simulink model "Kalman_Fliter"  (R2022b)
settings: Solver=VariableStepAuto  StartTime=0.0  StopTime=30  RelTol=1e-3
libraries: dspmathops x1
settings Model: Creator=zhouwenjie  LastModifiedBy=zhouwenjie

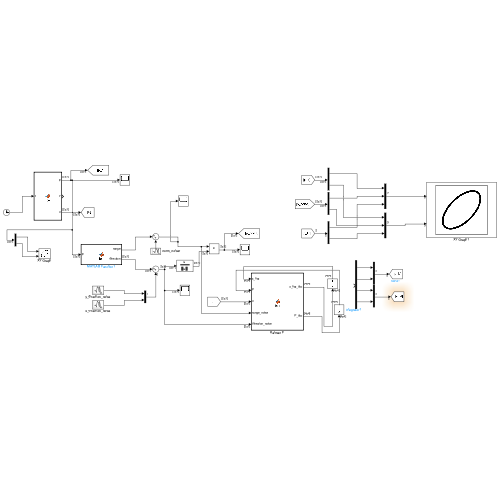
[thumbnail: Simulink's stored preview of the top-level diagram]
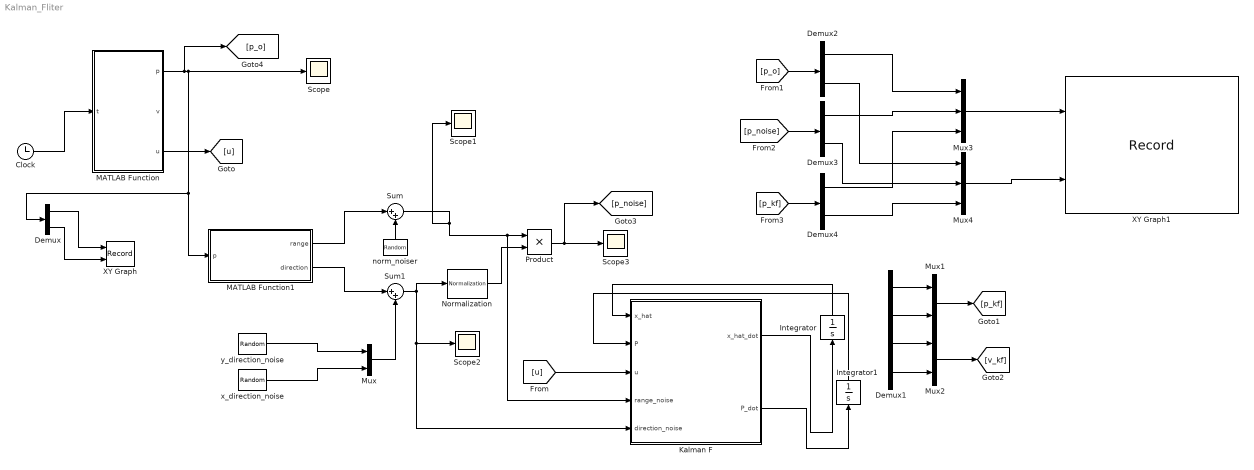
== system Kalman_Fliter ==
  Clock : Clock
  Demux{,2..4} (4 alike) : Demux  Outputs=2
  Demux1 : Demux
  Integrator : Integrator
  Integrator1 : Integrator
  Kalman F : MATLAB Function  TreatAsAtomicUnit=on
  MATLAB Function : MATLAB Function  TreatAsAtomicUnit=on
  MATLAB Function1 : MATLAB Function  TreatAsAtomicUnit=on
  Mux : Mux  Inputs=2
  Mux1 : Mux  Inputs=2
  Mux2 : Mux  Inputs=2
  Mux3 : Mux  Inputs=3
  Mux4 : Mux  Inputs=3
  Normalization : dspmathops/Normalization  NormType=2-norm  Bias=1e-10  NormOver=Each column  Dimension=1  roundingMode=Floor  overflowMode=off  accumDataTypeStr=Inherit: Same as product output  accumLastDataTypeStr=Inherit: Same as product output  outputDataTypeStr=Inherit: Same as product output  outputMin=[]  outputMax=[]  outputLastDataTypeStr=Inherit: Same as product output
  Product : Product
  Scope{,1..3} (4 alike) : Scope
  Sum : Sum  Inputs=|++
  Sum1 : Sum  Inputs=|++
  XY Graph : Record  FileSettingsInternal="{\"entries\":[{\"content\":{\"excelSettings\":{\"content\":{},\"type\":\"Streamout.ExcelSettings\"}},\"type\":\"Streamout.FileSettingStorage\",\"uuid\":\"d119d5ed-e209-42ba-8edb-009befcb7634\"}],\"packageUris\":[\"http://schema.mathworks.com/mf0/streamout_blocks/R2020a\"],\"version\":\"1.0\"}"  Layout=[1 1]  SignalsInternal="{\"entries\":[{\"content\":{\"signals\":[{\"content\":{\"blockPath\":[\"Kalman_Fliter/XY Graph\"],\"channel\":[],\"dimensions\":[1,1],\"domain\":\"Kalman_Fliter/XY Graph\",\"lineColor\":\"#a2142f\",\"plots\":[1],\"port\":1,\"sid\":[\"\"],\"signalID\":563,\"signalName\":\"Demux:1\"},\"type\":\"RecordBlkView.Signal\",\"uuid\":\"1961980f-dccb-4910-a77f-37722e977325\"},{\"content\":{\"blockPath\":[\"Kalman_Fliter/XY Graph\"],\"channel\":[],\"dimensions\":[1,1],\"domain\":\"Kalman_Fliter/XY Graph\",\"lineColor\":\"#139fff\",\"plots\":[1],\"port\":2,\"sid\":[\"\"],\"signalID\":567,\"signalName\":\"Demux:2\"},\"type\":\"RecordBlkView.Signal\",\"uuid\":\"f8809605-92a7-48fe-8c9b-7ed229beba8b\"}]},\"type\":\"RecordBlkView.InputSignals\",\"uuid\":\"e8c07406-b687-4a26-805d-c1320ae853b1\"}],\"packageUris\":[\"http://schema.mathworks.com/mf0/streamout_blocks/R2020a\"],\"version\":\"1.0\"}"  VisualizationBindings="{\"xyplotplugin\":{\"info\":[{\"series\":[{\"bindingParametersList\":[{\"parameter\":\"X-Axis\",\"signalID\":563,\"signalName\":\"Demux:1\"},{\"parameter\":\"Y-Axis\",\"signalID\":567,\"signalName\":\"Demux:2\"}],\"seriesID\":503},{\"bindingParametersList\":[{\"parameter\":\"Y-Axis\",\"signalID\":567,\"signalName\":\"Demux:2\"},{\"parameter\":\"X-Axis\",\"signalID\":563,\"signalName\":\"Demux:1\"}],\"seriesID\":363}],\"subplotID\":1}]}}"  CompatibilityTag=XY
  XY Graph1 : Record  FileSettingsInternal="{\"entries\":[{\"content\":{\"excelSettings\":{\"content\":{},\"type\":\"Streamout.ExcelSettings\"}},\"type\":\"Streamout.FileSettingStorage\",\"uuid\":\"eefeb38a-37b1-42c2-865b-dc8e865e0e60\"}],\"packageUris\":[\"http://schema.mathworks.com/mf0/streamout_blocks/R2020a\"],\"version\":\"1.0\"}"  Layout=[1 1]  SignalsInternal="{\"entries\":[{\"content\":{\"signals\":[{\"content\":{\"blockPath\":[\"Kalman_Fliter/XY Graph1\"],\"channel\":[],\"dimensions\":[3],\"domain\":\"Kalman_Fliter/XY Graph1\",\"hasChildren\":true,\"lineColor\":\"#64d413\",\"plots\":[],\"port\":1,\"sid\":[\"\"],\"signalID\":571,\"signalName\":\"Mux3\"},\"type\":\"RecordBlkView.Signal\",\"uuid\":\"0d81fedb-c315-4810-a6c0-24634af0a88d\"},{\"content\":{\"blockPath\":[\"Kalman_Fliter/XY Graph1\"],\"channel\":[1],\"dimensions\":[3],\"domain\":\"Kalman_Fliter/XY Graph1\",\"lineColor\":\"#d95319\",\"parentID\":571,\"plots\":[],\"port\":1,\"sid\":[\"\"],\"signalID\":572,\"signalName\":\"Mux3\"},\"type\":\"RecordBlkView.Signal\",\"uuid\":\"11839326-3698-4c45-9993-6f57091d2d65\"},{\"content\":{\"blockPath\":[\"Kalman_Fliter/XY Graph1\"],\"channel\":[],\"dimensions\":[3],\"domain\":\"Kalman_Fliter/XY Graph1\",\"hasChildren\":true,\"lineColor\":\"#fe330a\",\"plots\":[],\"port\":2,\"sid\":[\"\"],\"signalID\":576,\"signalName\":\"Mux4\"},\"type\":\"RecordBlkView.Signal\",\"uuid\":\"38af830b-27b1-40c6-b5d0-badb30e50f9a\"},{\"content\":{\"blockPath\":[\"Kalman_Fliter/XY Graph1\"],\"channel\":[1],\"dimensions\":[3],\"domain\":\"Kalman_Fliter/XY Graph1\",\"lineColor\":\"#7e2f8e\",\"parentID\":576,\"plots\":[],\"port\":2,\"sid\":[\"\"],\"signalID\":577,\"signalName\":\"Mux4\"},\"type\":\"RecordBlkView.Signal\",\"uuid\":\"8c4516df-ef14-4136-9417-f3e6a420cddc\"},{\"content\":{\"blockPath\":[\"Kalman_Fliter/XY Graph1\"],\"channel\":[2],\"dimensions\":[3],\"domain\":\"Kalman_Fliter/XY Graph1\",\"lineColor\":\"#77ac30\",\"parentID\":571,\"plots\":[],\"port\":1,\"sid\":[\"\"],\"signalID\":581,\"signalName\":\"Mux3\"},\"type\":\"RecordBlkView.Signal\",\"uuid\":\"d887d16f-7e2d-4d86-99dc-17678c9a946d\"},{\"content\":{\"blockPath\":[\"Kalman_Fliter/XY Graph1\"],\"channel\":[3],\"dimensions\":[3],\"domain\":\"Kalman_Fliter/XY Graph1\",\"lineColor\":\"#4dbeee\",\"parentID\":571,\"plots\":[],\"port\":1,\"sid\":[\"\"],\"signalID\":582,\"signalName\":\"Mux3\"},\"type\":\"RecordBlkView.Signal\",\"uuid\":\"1185f293-7a12-4181-bfa4-f7e996d1777d\"},{\"content\":{\"blockPath\":[\"Kalman_Fliter/XY Graph1\"],\"channel\":[2],\"dimensions\":[3],\"domain\":\"Kalman_Fliter/XY Graph1\",\"lineColor\":\"#a2142f\",\"parentID\":576,\"plots\":[],\"port\":2,\"sid\":[\"\"],\"signalID\":583,\"signalName\":\"Mux4\"},\"type\":\"RecordBlkView.Signal\",\"uuid\":\"4d6cb4ea-8538-4e3f-b0d2-57ebaadc180e\"},{\"content\":{\"blockPath\":[\"Kalman_Fliter/XY Graph1\"],\"channel\":[3],\"dimensions\":[3],\"domain\":\"Kalman_Fliter/XY Graph1\",\"lineColor\":\"#139fff\",\"parentID\":576,\"plots\":[],\"port\":2,\"sid\":[\"\"],\"signalID\":584,\"signalName\":\"Mux4\"},\"type\":\"RecordBlkView.Signal\",\"uuid\":\"043a01ad-2742-4b7c-882e-cd2255d83c8f\"}]},\"type\":\"RecordBlkView.InputSignals\",\"uuid\":\"c6b6343b-feff-4232-9459-ff0579f05e53\"}],\"packageUris\":[\"http://schema.mathworks.com/mf0/streamout_blocks/R2020a\"],\"version\":\"1.0\"}"  VisualizationBindings="{\"xyplotplugin\":{\"info\":[{\"series\":[],\"subplotID\":1}]}}"  CompatibilityTag=XY
  norm_noiser : RandomNumber  Variance=0.001  SampleTime=0.005
  x_direction_noise : RandomNumber  Variance=0.001  SampleTime=0.005
  y_direction_noise : RandomNumber  Variance=0.001  SampleTime=0.005
  wires:
  Clock/1 -> MATLAB Function/1(t)
  MATLAB Function/1(p) -> [p_o], Demux/1, MATLAB Function1/1(p), Scope/1
  norm_noiser/1 -> Sum/2
  MATLAB Function1/1(range) -> Sum/1
  Sum/1 -> Scope1/1, Kalman F/4(range_noise), Product/1
  MATLAB Function1/2(direction) -> Sum1/1
  y_direction_noise/1 -> Mux/1
  x_direction_noise/1 -> Mux/2
  Mux/1 -> Sum1/2
  Sum1/1 -> Normalization/1, Kalman F/5(direction_noise), Scope2/1
  Demux/1 -> XY Graph/1
  Demux/2 -> XY Graph/2
  Product/1 -> [p_noise], Scope3/1
  Normalization/1 -> Product/2
  [u] -> Kalman F/3(u)
  MATLAB Function/3(u) -> [u]
  Kalman F/2(P_dot) -> Integrator1/1
  Kalman F/1(x_hat_dot) -> Integrator/1
  Integrator1/1 -> Kalman F/2(P)
  Integrator/1 -> Kalman F/1(x_hat)
  Demux1/1 -> Mux1/1
  Demux1/2 -> Mux1/2
  Demux1/4 -> Mux2/2
  Demux1/3 -> Mux2/1
  Mux1/1 -> [p_kf]
  Mux2/1 -> [v_kf]
  Mux3/1 -> XY Graph1/1
  Mux4/1 -> XY Graph1/2
  [p_o] -> Demux2/1
  [p_kf] -> Demux4/1
  [p_noise] -> Demux3/1
  Demux2/1 -> Mux3/1
  Demux3/1 -> Mux3/2
  Demux4/1 -> Mux3/3
  Demux2/2 -> Mux4/1
  Demux3/2 -> Mux4/2
  Demux4/2 -> Mux4/3

== matlab function Kalman_Fliter/MATLAB Function1 ==
  data: p input; range output; direction output
function [range,direction]  = fcn(p)

range = norm(p);
direction = p/range;

== matlab function Kalman_Fliter/MATLAB Function ==
  data: t input; p output; v output; u output
function [p,v,u]  = fcn(t)

a = 1;
b = 1;
alpha = 1;
beta = 1;

p = [a*cos(alpha*t);
    b*sin(beta*t)];


v = [-a*alpha*sin(alpha*t);
     b*beta*cos(beta*t)];

u = [-a*alpha^2*cos(alpha*t);
     -b*beta^2*sin(beta*t)];

== matlab function Kalman_Fliter/Kalman F ==
  data: x_hat input; x_hat_dot output; P_dot output; P input; u input; range_noise input; direction_noise input
function [x_hat_dot, P_dot] = fcn(x_hat, P, u, range_noise,direction_noise)
% 状态转移矩阵
A = [zeros(2), eye(2);
     zeros(2), zeros(2)];
%control martix

% 观测矩阵
C = [eye(2), zeros(2)];

% 状态噪声协方差矩阵
Q = 1e-7*eye(4);

% 测量噪声协方差矩阵
R = 10*eye(2);

y = range_noise*direction_noise;
%Kalman Gain (simplfy C * P * C')the complete formula is K = P * C' * inv(C * P * C' + R)
K = P*C'/R;
%kalamn 修正后的状态空间方程
x_hat_dot = A*x_hat + [zeros(2,1); u] + K*(y - C*x_hat);
%误差协方差
P_dot = A*P + P*A' + Q - K*R*K';
